simulink subsystem "test"  (R2023b)
settings: Solver=VariableStepAuto  StartTime=0.0  StopTime=10.0  RelTol=1e-3
model mask{k1=0, k2=0, k3=0}
  mask prompts: k1 "Постоянное воздействие"; k2 "Синусоидальное воздействие"; k3 "Импульсное  воздействие"
settings Model: Creator=diontep  LastModifiedBy=lizar

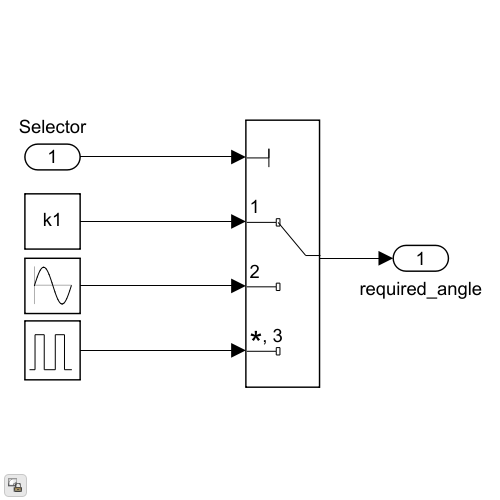
[thumbnail: Simulink's stored preview of the top-level diagram]
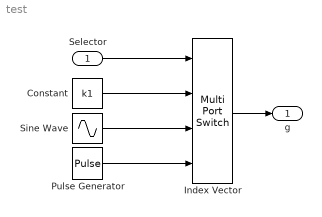
== system test ==
  Selector : Inport
  Constant : Constant  Value=k1
  Index Vector : MultiPortSwitch  SaturateOnIntegerOverflow=off  InputSameDT=off
  Pulse Generator : DiscretePulseGenerator  PulseType=Time based  Amplitude=k3  Period=10  PulseWidth=5
  Sine Wave : Sin  Amplitude=k2  SampleTime=0
  g : Outport
  wires:
  Index Vector/1 -> g/1
  Sine Wave/1 -> Index Vector/3
  Selector/1 -> Index Vector/1
  Constant/1 -> Index Vector/2
  Pulse Generator/1 -> Index Vector/4
